simulink model "Six_Phase_PWM"  (R2024a)
settings: Solver=FixedStepAuto  StartTime=0.0  StopTime=0.02  FixedStep=1e-6  RelTol=1e-3
libraries: simulink x1
settings Model: Creator=Ketan  LastModifiedBy=Ketan

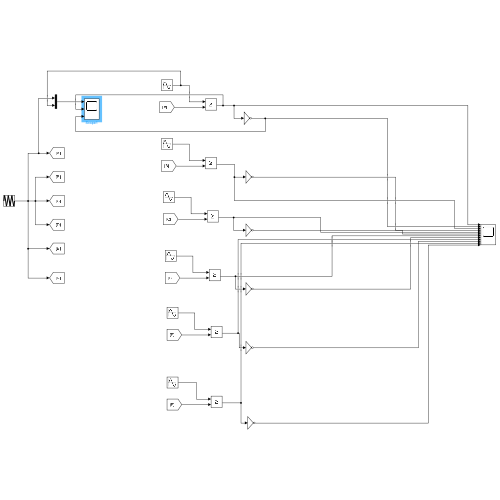
[thumbnail: Simulink's stored preview of the top-level diagram]
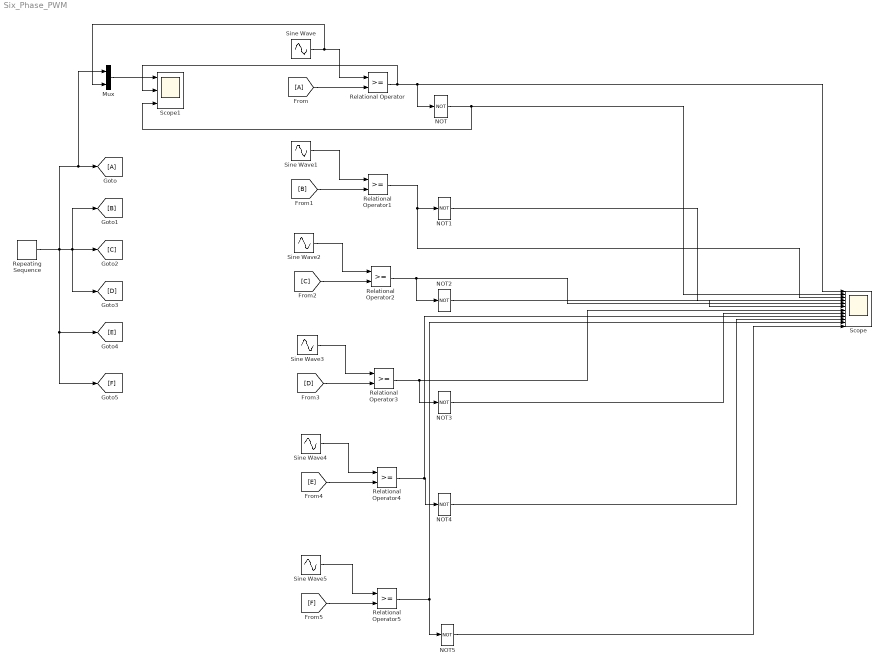
== system Six_Phase_PWM ==
  From : From
  Goto : Goto
  Mux : Mux  Inputs=2
  NOT{,1..5} (6 alike) : Logic  Operator=NOT  IconShape=distinctive  AllPortsSameDT=off  OutDataTypeStr=boolean
  Relational Operator{,1..5} (6 alike) : RelationalOperator  OutDataTypeStr=boolean  RndMeth=Simplest  InputSameDT=off
  Repeating Sequence : simulink/Sources/Repeating Sequence  rep_seq_t=[0 0.25 0.5 0.75 1]*(1/5000)  rep_seq_y=[0 1 0 -1 0]
  Scope : Scope  NumInputPorts=12
  Scope1 : Scope  NumInputPorts=3
  Sine Wave : Sin  Amplitude=0.9  Frequency=2*pi*50  SampleTime=0
  Sine Wave1 : Sin  Amplitude=0.9  Frequency=2*pi*50  Phase=pi/3  SampleTime=0
  Sine Wave2 : Sin  Amplitude=0.9  Frequency=2*pi*50  Phase=(2*pi)/3  SampleTime=0
  Sine Wave3 : Sin  Amplitude=0.9  Frequency=2*pi*50  Phase=(3*pi)/3  SampleTime=0
  Sine Wave4 : Sin  Amplitude=0.9  Frequency=2*pi*50  Phase=(4*pi)/3  SampleTime=0
  Sine Wave5 : Sin  Amplitude=0.9  Frequency=2*pi*50  Phase=(5*pi)/3  SampleTime=0
  wires:
  NOT3/1 -> Scope/8
  NOT2/1 -> Scope/6
  NOT/1 -> Scope1/3, Scope/2
  [E] -> Relational Operator4/2
  Sine Wave4/1 -> Relational Operator4/1
  Relational Operator/1 -> Scope1/2, Scope/1, NOT/1
  NOT4/1 -> Scope/10
  Sine Wave1/1 -> Relational Operator1/1
  Relational Operator3/1 -> Scope/7, NOT3/1
  Relational Operator1/1 -> Scope/3, NOT1/1
  Sine Wave2/1 -> Relational Operator2/1
  Repeating Sequence/1 -> [F], [E], Mux/1, Goto/1, [D], [B], [C]
  [D] -> Relational Operator3/2
  From/1 -> Relational Operator/2
  Sine Wave/1 -> Mux/2, Relational Operator/1
  Relational Operator2/1 -> Scope/5, NOT2/1
  [C] -> Relational Operator2/2
  [B] -> Relational Operator1/2
  NOT1/1 -> Scope/4
  Relational Operator4/1 -> Scope/9, NOT4/1
  Sine Wave3/1 -> Relational Operator3/1
  Sine Wave5/1 -> Relational Operator5/1
  [F] -> Relational Operator5/2
  Relational Operator5/1 -> Scope/11, NOT5/1
  NOT5/1 -> Scope/12
  Mux/1 -> Scope1/1
